simulink model "NeuromuscularModel_3R60_2D"  (R2019b)
settings: Solver=ode15s  StartTime=0.0  StopTime=30  MaxStep=.01  RelTol=1e-4  AbsTol=1e-6  EnableMultiTasking=on
values from neighbouring files (symbols this model uses):
  dt_visual = 1/50    (= 0.02)    [evaluateCost.m]    (also in evaluateCostCMG.m; optimize.m = 0.0333333333333; optimizeCMG.m; setVars.m = 0.0333333333333)
  initialTargetAngle = 70*pi/180    (= 1.2217304764)    [ControlParams.m]    (also in setInit.m)
  LongDelay = 0.020/2    (= 0.01)    [ControlParams.m]
  LongLoopDelay = 0.030    (= 0.03)    [ControlParams.m]
  LPreStimBFSHst = 0.02    [ControlParams.m]    (also in assignGains.m = Gains(51); assignGainsSagittal.m = GainsSagittal(51))
  LPreStimGASst = 0.01    [ControlParams.m]    (also in assignGains.m = Gains(52); assignGainsSagittal.m = GainsSagittal(52))
  LPreStimGLUst = 0.05    [ControlParams.m]    (also in assignGains.m = Gains(47); assignGainsSagittal.m = GainsSagittal(47))
  LPreStimHABst = 0.01    [ControlParams.m]
  LPreStimHADst = 0.01    [ControlParams.m]
  LPreStimHAMst = 0.05    [ControlParams.m]    (also in assignGains.m = Gains(48); assignGainsSagittal.m = GainsSagittal(48))
  LPreStimHFLst = 0.05    [ControlParams.m]    (also in assignGains.m = Gains(46); assignGainsSagittal.m = GainsSagittal(46))
  LPreStimRFst = 0.01    [ControlParams.m]    (also in assignGains.m = Gains(49); assignGainsSagittal.m = GainsSagittal(49))
  LPreStimSOLst = 0.01    [ControlParams.m]    (also in assignGains.m = Gains(53); assignGainsSagittal.m = GainsSagittal(53))
  LPreStimTAst = 0.01    [ControlParams.m]    (also in assignGains.m = Gains(54); assignGainsSagittal.m = GainsSagittal(54))
  LPreStimVASst = 0.08    [ControlParams.m]    (also in assignGains.m = Gains(50); assignGainsSagittal.m = GainsSagittal(50))
  MidDelay = 0.010/2    (= 0.005)    [ControlParams.m]
  RPreStimGLUsw = 0.01    [ControlParams.m]    (also in assignGains.m = Gains(95); assignGainsSagittal.m = GainsSagittal(94))
  RPreStimHABsw = 0.01    [ControlParams.m]
  RPreStimHADsw = 0.01    [ControlParams.m]
  RPreStimHAMsw = 0.01    [ControlParams.m]    (also in assignGains.m = Gains(96); assignGainsSagittal.m = GainsSagittal(95))
  RPreStimHFLsw = 0.01    [ControlParams.m]    (also in assignGains.m = Gains(94); assignGainsSagittal.m = GainsSagittal(93))
  RPreStimRFsw = 0.01    [ControlParams.m]    (also in assignGains.m = Gains(97); assignGainsSagittal.m = GainsSagittal(96))
  ShortDelay = 0.005/2    (= 0.0025)    [ControlParams.m]
  termination_height = 0.5    [ControlParams.m]
  thetaHATref = 0    [ControlParams.m]
  vy0 = paramIC(10)*.2    [setInit.m]
undefined symbols (not defined in the file or in its folder): g, hatLeftHipToCenterDistWidth, hatLeftHipToCG, initialTargetAngleR, magnitude, obstacle_depth, obstacle_height, obstacle_width, obstacle_x, X, Y, y0, Z
libraries: NeuroMuscularLibrary x101, sm_lib x24, nesl_utility x16, simulink x5
(part 1 of 5)
settings Model: SimulationMode=rapid-accelerator  ParamWorkspaceSource=ReferencedWorkspace  ExtModeTrigDuration=100  TunableVars=GainGAS,GainGLU,GainHAM,GainKneeOverExt,GainSOL,GainSOLTA,GainTA,GainVAS,Kglu,PosGainGG,SpeedGainGG,groundTheta,groundX,groundZ,hipDGain,hipPGain,kneeExtendGain,kneeFlexGain,kneeHoldGain1,kneeHoldGain2,kneeStopGain,legAngleFilter,legLengthClr,simbiconGainD,simbiconGainV,simbiconLegAngle0  TunableVarsStorageClass=Auto,Auto,Auto,Auto,Auto,Auto,Auto,Auto,Auto,Auto,Auto,Auto,Auto,Auto,Auto,Auto,Auto,Auto,Auto,Auto,Auto,Auto,Auto,Auto,Auto,Auto  TunableVarsTypeQualifier=,,,,,,,,,,,,,,,,,,,,,,,,,  Creator=nitisht  LastModifiedBy=Nathan
settings SolverCC: AutoScaleAbsTol=off  ZeroCrossAlgorithm=Adaptive
settings DataIOCC: LimitDataPoints=on  SaveFinalState=on  SaveFormat=StructureWithTime  SaveOutput=off  SaveState=on  ReturnWorkspaceOutputs=off  StateSaveName=tmp_raccel_xout  SignalLoggingName=tmp_raccel_logsout
settings OptimizationCC: DefaultParameterBehavior=Inlined  EfficientMapNaN2IntZero=off  LifeSpan=inf  SimCompilerOptimization=on  AccelVerboseBuild=on
settings DebuggingCC: SaveWithDisabledLinksMsg=none  UnderspecifiedInitializationDetection=Classic  MergeDetectMultiDrivingBlocksExec=none  IgnoredZcDiagnostic=none  SolverPrmCheckMsg=warning  StateNameClashWarn=warning  SFUnexpectedBacktrackingDiag=warning  SFNoUnconditionalDefaultTransitionDiag=warning  SFExecutionAtInitializationDiag=none  ArithmeticOperatorsInVariantConditions=warning
settings HardwareCC: ProdBitPerPointer=32  ProdBitPerSizeT=32  ProdBitPerPtrDiffT=32  ProdLargestAtomicFloat=None  ProdIntDivRoundTo=Undefined  ProdEndianess=Unspecified  ProdWordSize=32  ProdHWDeviceType=Generic->Unspecified (assume 32-bit Generic)  TargetBitPerPointer=64  TargetBitPerSizeT=64  TargetBitPerPtrDiffT=64  TargetLongLongMode=on  TargetIntDivRoundTo=Zero  TargetEndianess=LittleEndian  TargetWordSize=64  TargetHWDeviceType=MATLAB Host  ProdEqTarget=off
settings ModelReferenceCC: PropagateSignalLabelsOutOfModel=off
settings SFSimCC: SFSimEcho=off  SimUseLocalCustomCode=off  CustomCodeUndefinedFunction=UseInterfaceOnly
settings RTWCC: SystemTargetFile=raccel.tlc  TemplateMakefile=raccel_default_tmf  RTWUseLocalCustomCode=off  RTWUseSimCustomCode=on
settings CodeAppCC: GenerateComments=off  MaxIdLength=128  MangleLength=10  SimulinkBlockComments=off
settings RaccelTargetCC: GeneratePreprocessorConditionals=Disable all  MultiInstanceERTCode=off  PreserveStateflowLocalDataDimensions=off  ENABLE_SLEXEC_SSBRIDGE=0  RTWCAPIParams=off
settings ConfigComp: CovMetricSettings=dw  CovHtmlReporting=on  CovSaveCumulativeToWorkspaceVar=on  CovSaveSingleToWorkspaceVar=on  CovExternalEMLEnable=off  CovSFcnEnable=off
settings SimscapeCC: SimscapeNormalizeSystem=off
settings ConfigurationSet: Description=SimMechanics 2G
settings ExplorerConfigSet: InternalSimMechanicsExplorerSettings="<ExplorerConfiguration><canonicalview>default</canonicalview><AnimationSetting><BasePlaybackSpeed>1.0</BasePlaybackSpeed><PlaybackSpeedFactor>1.0</PlaybackSpeedFactor></AnimationSetting><TilePanel><TileInfo><Tiles Columns=\"1\" Count=\"1\" Rows=\"1\"><Column Weight=\"1\"/><Row Weight=\"1\"/><Tile Height=\"1\" Width=\"1\" X=\"0\" Y=\"0\"/></Tiles></TileInfo><SceneInfo><SceneViewer><BGColor><R>0.60000002384185791</R><G>0.60000002384185791</G><B>0.60000002384185791</B></BGColor><Camera><DoPerspective>on</DoPerspective><Position><X>-0.182248624365848877</X><Y>-2.44999999999999929</Y><Z>0.98448567525706232</Z></Position><Center><X>-0.182248624365848877</X><Y>-1.44999999999999929</Y><Z>0.98448567525706232</Z></Center><Up><X>0</X><Y>0</Y><Z>1</Z></Up><ViewLimDist>1</ViewLimDist><YLim>0.466307658154998583</YLim><XLim>0.945026546755187269</XLim></Camera></SceneViewer></SceneInfo></TilePanel><MechEditorPanel><Cameras><Camera><Id>Camera1</Id><Value><Name>Camera1</Name><NativeCamera><PositionTrackingFeature>Body_Mechanics_Layer.Whole_Body_Tracking_Camera.R</PositionTrackingFeature><CenterTrackingFeature>Body_Mechanics_Layer.World_Frame_X_forward_Y_lateral_Z_up1.W</CenterTrackingFeature><UpVectorTrackingFeature>Body_Mechanics_Layer.World_Frame_X_forward_Y_lateral_Z_up1.W</UpVectorTrackingFeature><CenterTrackingOrigin>off</CenterTrackingOrigin><CenterTrackingDirection>+Y</CenterTrackingDirection><UpVectorTrackingDirection>+Z</UpVectorTrackingDirection></NativeCamera></Value></Camera></Cameras><GfxPanelCameraMap><MapElement CameraMLId=\"Camera1\" GfxPanelIndex=\"0\"/></GfxPanelCameraMap><VideoCreator><PlaybackSpeedRatio>1.0</PlaybackSpeedRatio><FrameRate>30</FrameRate><VideoFormat>Motion JPEG AVI</VideoFormat><FrameSize>auto</FrameSize></VideoCreator></MechEditorPanel></ExplorerConfiguration>"

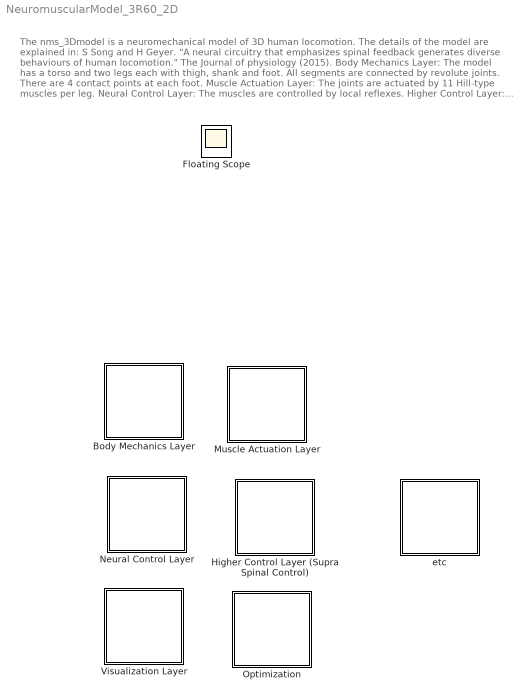
== system NeuromuscularModel_3R60_2D ==
  note: The nms_3Dmodel is a neuromechanical model of 3D human locomotion.
      | The details of the model are explained in:
      | S Song and H Geyer. "A neural circuitry that emphasizes spinal feedback
      | generates diverse behaviours of human locomotion." The Journal of physiology (2015).
      |
      | Body Mechanics Layer:
      | The model has a torso and two legs each with thigh, shank and foot.
      | All segments are connected by revolute joints.
      | There are 4 contact points at each foot.
      |
      | Muscle Actuation Layer:
      | The joints are actuated by 11 Hill-type muscles per leg.
      |
      | Neural Control Layer:
      | The muscles are controlled by local reflexes.
      |
      | Higher Control Layer:
      | The reflex pathways are modulated by the higher layer control.
  Body Mechanics Layer : Subsystem
  Higher Control Layer (Supra Spinal Control) : Subsystem
  Muscle Actuation Layer : Subsystem
  Neural Control Layer : Subsystem
  Optimization : Subsystem
  Visualization Layer : Subsystem
  etc : Subsystem
  Floating Scope : Scope
